simulink library "INT_WESDem_SelectParam"  (R2016b)
settings: Solver=VariableStepAuto  StartTime=0.0  StopTime=10.0  RelTol=1e-3
settings Model: Creator=zhoukai  LastModifiedBy=zhoukai

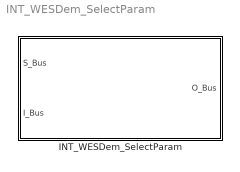
== system INT_WESDem_SelectParam ==
  INT_WESDem_SelectParam : Subsystem

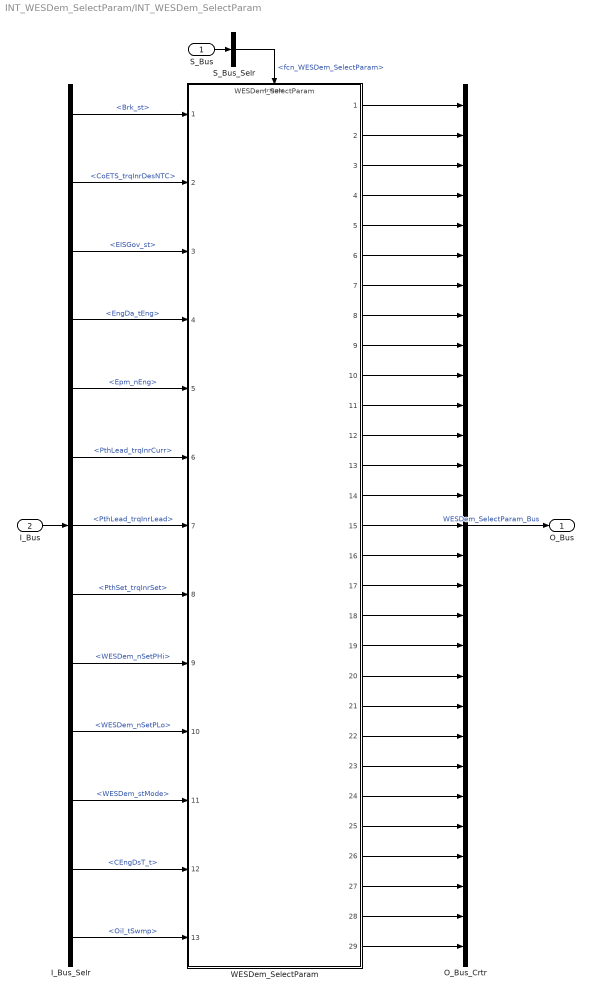
== system INT_WESDem_SelectParam/INT_WESDem_SelectParam ==
  S_Bus : Inport
  I_Bus : Inport  Port=2
  I_Bus_Selr : BusSelector  OutputSignals=Brk_st,CoETS_trqInrDesNTC,EISGov_st,EngDa_tEng,Epm_nEng,PthLead_trqInrCurr,PthLead_trqInrLead,PthSet_trqInrSet,WESDem_nSetPHi,WESDem_nSetPLo,WESDem_stMode,CEngDsT_t,Oil_tSwmp
  O_Bus_Crtr : BusCreator  Inputs=29
  S_Bus_Selr : BusSelector  OutputSignals=fcn_WESDem_SelectParam
  WESDem_SelectParam : ModelReference  ModelNameDialog=WESDem_SelectParam  SimulationMode=Normal  ModelReferenceVersion=1.52  TriggerPortName=function  TriggerPortTriggerType=function-call  TriggerPortStatesWhenEnabling=held
  O_Bus : Outport
  wires:
  S_Bus_Selr/1 -> WESDem_SelectParam/Trigger  "<fcn_WESDem_SelectParam>"
  S_Bus/1 -> S_Bus_Selr/1
  I_Bus/1 -> I_Bus_Selr/1
  I_Bus_Selr/1 -> WESDem_SelectParam/1  "<Brk_st>"
  I_Bus_Selr/2 -> WESDem_SelectParam/2  "<CoETS_trqInrDesNTC>"
  I_Bus_Selr/3 -> WESDem_SelectParam/3  "<EISGov_st>"
  I_Bus_Selr/4 -> WESDem_SelectParam/4  "<EngDa_tEng>"
  I_Bus_Selr/5 -> WESDem_SelectParam/5  "<Epm_nEng>"
  I_Bus_Selr/6 -> WESDem_SelectParam/6  "<PthLead_trqInrCurr>"
  I_Bus_Selr/7 -> WESDem_SelectParam/7  "<PthLead_trqInrLead>"
  I_Bus_Selr/8 -> WESDem_SelectParam/8  "<PthSet_trqInrSet>"
  I_Bus_Selr/9 -> WESDem_SelectParam/9  "<WESDem_nSetPHi>"
  I_Bus_Selr/10 -> WESDem_SelectParam/10  "<WESDem_nSetPLo>"
  I_Bus_Selr/11 -> WESDem_SelectParam/11  "<WESDem_stMode>"
  I_Bus_Selr/12 -> WESDem_SelectParam/12  "<CEngDsT_t>"
  I_Bus_Selr/13 -> WESDem_SelectParam/13  "<Oil_tSwmp>"
  O_Bus_Crtr/1 -> O_Bus/1  "WESDem_SelectParam_Bus"
  WESDem_SelectParam/1 -> O_Bus_Crtr/1
  WESDem_SelectParam/2 -> O_Bus_Crtr/2
  WESDem_SelectParam/3 -> O_Bus_Crtr/3
  WESDem_SelectParam/4 -> O_Bus_Crtr/4
  WESDem_SelectParam/5 -> O_Bus_Crtr/5
  WESDem_SelectParam/6 -> O_Bus_Crtr/6
  WESDem_SelectParam/7 -> O_Bus_Crtr/7
  WESDem_SelectParam/8 -> O_Bus_Crtr/8
  WESDem_SelectParam/9 -> O_Bus_Crtr/9
  WESDem_SelectParam/10 -> O_Bus_Crtr/10
  WESDem_SelectParam/11 -> O_Bus_Crtr/11
  WESDem_SelectParam/12 -> O_Bus_Crtr/12
  WESDem_SelectParam/13 -> O_Bus_Crtr/13
  WESDem_SelectParam/14 -> O_Bus_Crtr/14
  WESDem_SelectParam/15 -> O_Bus_Crtr/15
  WESDem_SelectParam/16 -> O_Bus_Crtr/16
  WESDem_SelectParam/17 -> O_Bus_Crtr/17
  WESDem_SelectParam/18 -> O_Bus_Crtr/18
  WESDem_SelectParam/19 -> O_Bus_Crtr/19
  WESDem_SelectParam/20 -> O_Bus_Crtr/20
  WESDem_SelectParam/21 -> O_Bus_Crtr/21
  WESDem_SelectParam/22 -> O_Bus_Crtr/22
  WESDem_SelectParam/23 -> O_Bus_Crtr/23
  WESDem_SelectParam/24 -> O_Bus_Crtr/24
  WESDem_SelectParam/25 -> O_Bus_Crtr/25
  WESDem_SelectParam/26 -> O_Bus_Crtr/26
  WESDem_SelectParam/27 -> O_Bus_Crtr/27
  WESDem_SelectParam/28 -> O_Bus_Crtr/28
  WESDem_SelectParam/29 -> O_Bus_Crtr/29
